simulink model "summerControlledGroup8"  (R2023b)
settings: Solver=VariableStepAuto  StartTime=0.0  StopTime=49860  RelTol=1e-3
undefined symbols (not defined in the file): J, Kd, Ke, Ks, Kt, La, Ra
libraries: slpidlib x2, simulink_extras x1
settings Model: Creator=jmars  LastModifiedBy=jmars
settings DataIOCC: ExternalInput=[dec_time dec_azimuth dec_altitude]  LoadExternalInput=on

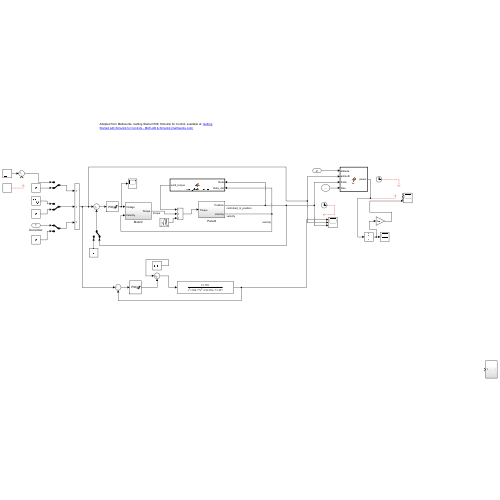
[thumbnail: Simulink's stored preview of the top-level diagram]
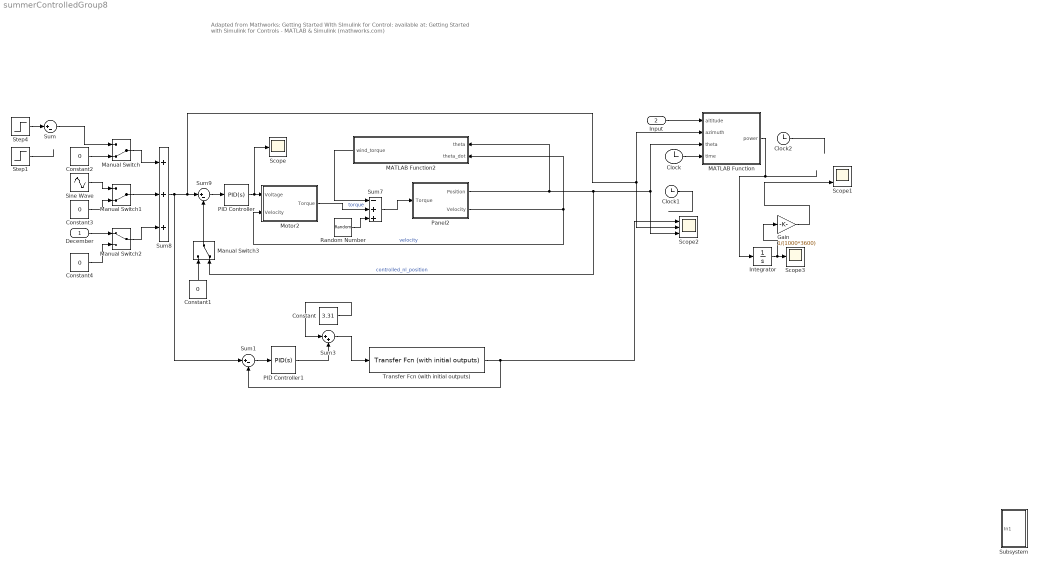
== system summerControlledGroup8 ==
  note: Adapted from Mathworks: Getting Started WIth SImulink for Control: available at: Getting Started with Simulink for Controls - MATLAB & Simulink (mathworks.com)
  December : Inport
  Input : Inport  Port=2
  Clock : Clock
  Clock1 : Clock
  Clock2 : Clock
      settings: Decimation=5
  Constant : Constant  Value=3.31  OutMin=[0]
  Constant{1..4} (4 alike) : Constant  Value=0
  Gain : Gain  Gain=1/(1000*3600)
  Integrator : Integrator
  MATLAB Function : MATLAB Function  TreatAsAtomicUnit=on
  MATLAB Function2 : MATLAB Function  TreatAsAtomicUnit=on
  Manual Switch : ManualSwitch  CurrentSetting=0
  Manual Switch1 : ManualSwitch  CurrentSetting=0
  Manual Switch2 : ManualSwitch
  Manual Switch3 : ManualSwitch  CurrentSetting=0
  Motor2 : Subsystem
  PID Controller : slpidlib/PID Controller  Controller=PID  Form=Parallel  TimeDomain=Continuous-time  UseExternalTs=off  SampleTime=-1  IntegratorMethod=Forward Euler  FilterMethod=Forward Euler  ControllerParametersSource=internal  P=6141/100  I=2.535e4/100  UseKiTs=off  D=4.098e4/100  N=13.7703  UseFilter=on  TunerSelectOption=Transfer Function Based (PID Tuner App)  InitialConditionSource=internal  InitialConditionForIntegrator=0  InitialConditionForFilter=0  DifferentiatorICPrevScaledInput=0  ExternalReset=none  TrackingMode=off  Kt=1  LimitOutput=on  SatLimitsSource=internal  UpperSaturationLimit=27.5  LowerSaturationLimit=-27.5  LinearizeAsGain=on  AntiWindupMode=none  Kb=1  LimitIntegrator=off  UpperIntegratorSaturationLimit=inf  LowerIntegratorSaturationLimit=-inf  POutMin=[]  POutMax=[]  IOutMin=[]  IOutMax=[]  DOutMin=[]  DOutMax=[]  NOutMin=[]  NOutMax=[]  SumOutMin=[]  SumOutMax=[]  SaturationOutMin=[]  SaturationOutMax=[]  PParamMin=[]  PParamMax=[]  IParamMin=[]  IParamMax=[]  DParamMin=[]  DParamMax=[]  NParamMin=[]  NParamMax=[]  KbParamMin=[]  KbParamMax=[]  KtParamMin=[]  KtParamMax=[]  KbOutMin=[]  KbOutMax=[]  KtOutMin=[]  KtOutMax=[]  IntegratorOutMin=[]  IntegratorOutMax=[]  FilterOutMin=[]  FilterOutMax=[]  SumI1OutMin=[]  SumI1OutMax=[]  SumI2OutMin=[]  SumI2OutMax=[]  SumI3OutMin=[]  SumI3OutMax=[]  SumI4OutMin=[]  SumI4OutMax=[]  SumDOutMin=[]  SumDOutMax=[]  DifferentiatorOutMin=[]  DifferentiatorOutMax=[]  FilterDiffOutCoefMin=[]  FilterDiffOutCoefMax=[]  ReciprocalOutMin=[]  ReciprocalOutMax=[]  SumDenOutMin=[]  SumDenOutMax=[]  SumNumOutMin=[]  SumNumOutMax=[]  DivideOutMin=[]  DivideOutMax=[]  UdiffTsProdOutMin=[]  UdiffTsProdOutMax=[]  NTsProdOutMin=[]  NTsProdOutMax=[]  UintegralTsProdOutMin=[]  UintegralTsProdOutMax=[]  UngainTsProdOutMin=[]  UngainTsProdOutMax=[]  ClampingZeroOutDataTypeStr=Inherit: Inherit via back propagation  ClampingZeroOutMin=[]  ClampingZeroOutMax=[]  FilterDenConstantOutDataTypeStr=Inherit: Inherit via back propagation  FilterDenConstantOutMin=[]  FilterDenConstantOutMax=[]  PCopyOutDataTypeStr=Inherit: Inherit via back propagation  PCopyOutMin=[]  PCopyOutMax=[]  NCopyOutDataTypeStr=Inherit: Inherit via back propagation  NCopyOutMin=[]  NCopyOutMax=[]  IntegratorContinuousStateAttributes=''  IntegratorStateMustResolveToSignalObject=off  IntegratorRTWStateStorageClass=Auto  FilterContinuousStateAttributes=''  FilterStateMustResolveToSignalObject=off  FilterRTWStateStorageClass=Auto  ParallelPVariant=InternalParameters  IdealPVariant=Disabled  IVariant=InternalParameters  DVariant=InternalParameters  IntegratorVariant=Continuous  SatVariant=Enabled  AWVariant=Passthrough  PCopyVariant=Disabled  TRVariant=Disabled  FdbkBlocksVariant=Forward  IdealPFdbkVariant=Disabled  SatFdbkVariant=Disabled  DerivativeFilterVariant=ContFilter  NVariant=InternalParameters  NCopyVariant=Disabled  FilterICVariant=InternalICsFilter  IntegratorICVariant=InternalICs  ExternalResetVariant=Disabled  TRSumVariant=Passthrough  SumFdbkVariant=Disabled  SumVariant=Sum_PID  TsampFilterVariant=InternalTs  TsampNgainVariant=Passthrough  TsampIntegralVariant=Disabled_SignalSpec  ExternalSaturationOutDataTypeStr=Inherit: Same as second input
  PID Controller1 : slpidlib/PID Controller  Controller=PID  Form=Parallel  TimeDomain=Continuous-time  UseExternalTs=off  SampleTime=-1  IntegratorMethod=Forward Euler  FilterMethod=Forward Euler  ControllerParametersSource=internal  P=6141/100  I=2.535e4/100  UseKiTs=off  D=4.098e4/100  N=13.7703  UseFilter=on  TunerSelectOption=Transfer Function Based (PID Tuner App)  InitialConditionSource=internal  InitialConditionForIntegrator=0  InitialConditionForFilter=0  DifferentiatorICPrevScaledInput=0  ExternalReset=none  TrackingMode=off  Kt=1  LimitOutput=on  SatLimitsSource=internal  UpperSaturationLimit=27.5  LowerSaturationLimit=-27.5  LinearizeAsGain=on  AntiWindupMode=none  Kb=1  LimitIntegrator=off  UpperIntegratorSaturationLimit=inf  LowerIntegratorSaturationLimit=-inf  POutMin=[]  POutMax=[]  IOutMin=[]  IOutMax=[]  DOutMin=[]  DOutMax=[]  NOutMin=[]  NOutMax=[]  SumOutMin=[]  SumOutMax=[]  SaturationOutMin=[]  SaturationOutMax=[]  PParamMin=[]  PParamMax=[]  IParamMin=[]  IParamMax=[]  DParamMin=[]  DParamMax=[]  NParamMin=[]  NParamMax=[]  KbParamMin=[]  KbParamMax=[]  KtParamMin=[]  KtParamMax=[]  KbOutMin=[]  KbOutMax=[]  KtOutMin=[]  KtOutMax=[]  IntegratorOutMin=[]  IntegratorOutMax=[]  FilterOutMin=[]  FilterOutMax=[]  SumI1OutMin=[]  SumI1OutMax=[]  SumI2OutMin=[]  SumI2OutMax=[]  SumI3OutMin=[]  SumI3OutMax=[]  SumI4OutMin=[]  SumI4OutMax=[]  SumDOutMin=[]  SumDOutMax=[]  DifferentiatorOutMin=[]  DifferentiatorOutMax=[]  FilterDiffOutCoefMin=[]  FilterDiffOutCoefMax=[]  ReciprocalOutMin=[]  ReciprocalOutMax=[]  SumDenOutMin=[]  SumDenOutMax=[]  SumNumOutMin=[]  SumNumOutMax=[]  DivideOutMin=[]  DivideOutMax=[]  UdiffTsProdOutMin=[]  UdiffTsProdOutMax=[]  NTsProdOutMin=[]  NTsProdOutMax=[]  UintegralTsProdOutMin=[]  UintegralTsProdOutMax=[]  UngainTsProdOutMin=[]  UngainTsProdOutMax=[]  ClampingZeroOutDataTypeStr=Inherit: Inherit via back propagation  ClampingZeroOutMin=[]  ClampingZeroOutMax=[]  FilterDenConstantOutDataTypeStr=Inherit: Inherit via back propagation  FilterDenConstantOutMin=[]  FilterDenConstantOutMax=[]  PCopyOutDataTypeStr=Inherit: Inherit via back propagation  PCopyOutMin=[]  PCopyOutMax=[]  NCopyOutDataTypeStr=Inherit: Inherit via back propagation  NCopyOutMin=[]  NCopyOutMax=[]  IntegratorContinuousStateAttributes=''  IntegratorStateMustResolveToSignalObject=off  IntegratorRTWStateStorageClass=Auto  FilterContinuousStateAttributes=''  FilterStateMustResolveToSignalObject=off  FilterRTWStateStorageClass=Auto  ParallelPVariant=InternalParameters  IdealPVariant=Disabled  IVariant=InternalParameters  DVariant=InternalParameters  IntegratorVariant=Continuous  SatVariant=Enabled  AWVariant=Passthrough  PCopyVariant=Disabled  TRVariant=Disabled  FdbkBlocksVariant=Forward  IdealPFdbkVariant=Disabled  SatFdbkVariant=Disabled  DerivativeFilterVariant=ContFilter  NVariant=InternalParameters  NCopyVariant=Disabled  FilterICVariant=InternalICsFilter  IntegratorICVariant=InternalICs  ExternalResetVariant=Disabled  TRSumVariant=Passthrough  SumFdbkVariant=Disabled  SumVariant=Sum_PID  TsampFilterVariant=InternalTs  TsampNgainVariant=Passthrough  TsampIntegralVariant=Disabled_SignalSpec  ExternalSaturationOutDataTypeStr=Inherit: Same as second input
  Panel2 : Subsystem
  Random Number : RandomNumber  Variance=0.01  SampleTime=10
  Scope : Scope
  Scope1 : Scope  NumInputPorts=3
  Scope2 : Scope  NumInputPorts=3
  Scope3 : Scope
  Sine Wave : Sin  Bias=1.1019  SampleTime=0
  Step1 : Step  Time=20  After=8.8981  SampleTime=0
  Step4 : Step  Time=10  Before=1.1019  After=10  SampleTime=0
  Subsystem : Subsystem
  Sum : Sum  Inputs=|+-
  Sum1 : Sum  Inputs=|+-
  Sum3 : Sum  Inputs=|++
  Sum7 : Sum  Inputs=-++
  Sum8 : Sum  Inputs=+++
  Sum9 : Sum  Inputs=|+-
  Transfer Fcn (with initial outputs) : simulink_extras/Additional Linear/Transfer Fcn (with initial outputs)  N=[23.7894]  D="[1  306.7708 182.0498 71.4275]"  Y0=1.1019  U0=3.31
  wires:
  Sine Wave/1 -> Manual Switch1/1
  Manual Switch2/1 -> Sum8/3
  Manual Switch1/1 -> Sum8/2
  Constant4/1 -> Manual Switch2/2
  Panel2/1(Position) -> Manual Switch3/2, Scope2/3, MATLAB Function/3(theta), MATLAB Function2/1(theta)  "controlled_nl_position"
  Sum7/1 -> Panel2/1(Torque)
  Sum8/1 -> Sum1/1, Scope2/2, MATLAB Function/2(azimuth), Sum9/1
  December/1 -> Manual Switch2/1
  Constant2/1 -> Manual Switch/2
  Sum9/1 -> PID Controller/1
  Manual Switch/1 -> Sum8/1
  Motor2/1(Torque) -> Sum7/2  "torque"
  Constant3/1 -> Manual Switch1/2
  MATLAB Function2/1(wind_torque) -> Sum7/1
  Panel2/2(Velocity) -> Motor2/2(Velocity), MATLAB Function2/2(theta_dot)  "velocity"
  Step4/1 -> Sum/1
  Sum/1 -> Manual Switch/1
  Step1/1 -> ?
  Manual Switch3/1 -> Sum9/2
  Constant1/1 -> Manual Switch3/1
  Sum1/1 -> PID Controller1/1
  Transfer Fcn (with initial outputs)/1 -> Scope2/1, Sum1/2
  PID Controller/1 -> Scope/1, Motor2/1(Voltage)
  Random Number/1 -> Sum7/3
  Input/1 -> MATLAB Function/1(altitude)
  Clock/1 -> MATLAB Function/4(time)
  MATLAB Function/1(power) -> Integrator/1
  Integrator/1 -> Gain/1, Scope3/1
  PID Controller1/1 -> Sum3/2
  Constant/1 -> Sum3/1
  Sum3/1 -> Transfer Fcn (with initial outputs)/1
  Clock1/1 -> ?
  Gain/1 -> Scope1/3
  Clock2/1 -> ?

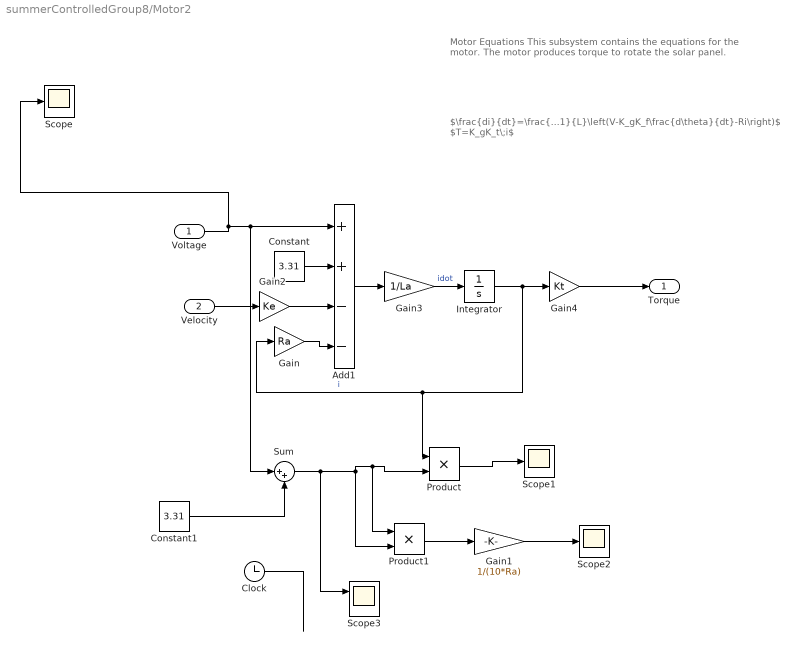
== system summerControlledGroup8/Motor2 ==
  note: $\frac{di}{dt}=\frac{1}{L}\left(V-K_gK_f\frac{d\theta}{dt}-Ri\right)$
      | $T=K_gK_t\;i$
  note: Motor Equations
      |
      | This subsystem contains the equations for the motor. The motor produces torque to rotate the solar panel.
  Voltage : Inport
  Velocity : Inport  Port=2
  Add1 : Sum  Inputs=++--
  Clock : Clock
      settings: Decimation=5
  Constant : Constant  Value=3.31  OutMin=[0]
  Constant1 : Constant  Value=3.31  OutMin=[0]
  Gain : Gain  Gain=Ra
  Gain1 : Gain  Gain=1/(10*Ra)
  Gain2 : Gain  Gain=Ke
  Gain3 : Gain  Gain=1/La
  Gain4 : Gain  Gain=Kt
  Integrator : Integrator  InitialCondition=3.5
  Product : Product
  Product1 : Product
  Scope : Scope
  Scope1 : Scope
  Scope2 : Scope
  Scope3 : Scope  NumInputPorts=2
  Sum : Sum  Inputs=|++
  Torque : Outport
  wires:
  Voltage/1 -> Scope/1, Sum/1, Add1/1
  Gain2/1 -> Add1/3
  Gain3/1 -> Integrator/1  "idot"
  Gain/1 -> Add1/4
  Integrator/1 -> Product/1, Gain/1, Gain4/1  "i"
  Add1/1 -> Gain3/1
  Velocity/1 -> Gain2/1
  Gain4/1 -> Torque/1
  Constant/1 -> Add1/2
  Product/1 -> Scope1/1
  Sum/1 -> Scope3/1, Product1/1, Product/2, Product1/2
  Constant1/1 -> Sum/2
  Product1/1 -> Gain1/1
  Gain1/1 -> Scope2/1
  Clock/1 -> ?

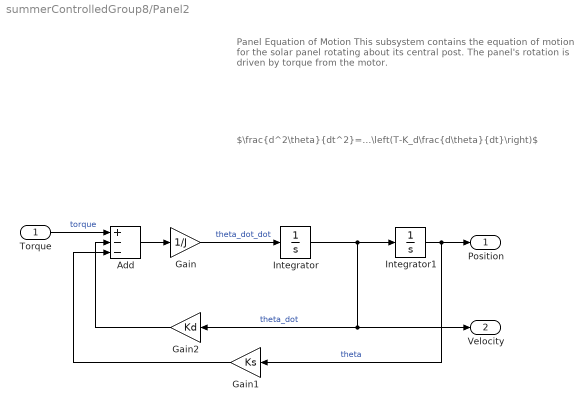
== system summerControlledGroup8/Panel2 ==
  note: $\frac{d^2\theta}{dt^2}=\frac{1}{J}\left(T-K_d\frac{d\theta}{dt}\right)$
  note: Panel Equation of Motion
      |
      | This subsystem contains the equation of motion for the solar panel rotating about its central post. The panel's rotation is driven by torque from the motor.
  Torque : Inport
  Add : Sum  Inputs=+--
  Gain : Gain  Gain=1/J
  Gain1 : Gain  Gain=Ks
  Gain2 : Gain  Gain=Kd
  Integrator : Integrator
  Integrator1 : Integrator  InitialCondition=1.1019
  Position : Outport
  Velocity : Outport  Port=2
  wires:
  Torque/1 -> Add/1  "torque"
  Add/1 -> Gain/1
  Integrator/1 -> Velocity/1, Gain2/1, Integrator1/1  "theta_dot"
  Gain2/1 -> Add/2
  Gain/1 -> Integrator/1  "theta_dot_dot"
  Integrator1/1 -> Gain1/1, Position/1  "theta"
  Gain1/1 -> Add/3

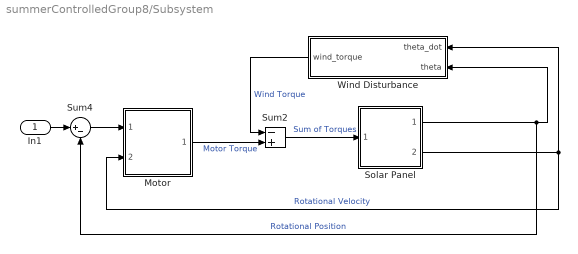
== system summerControlledGroup8/Subsystem ==
  In1 : Inport
  Motor : Subsystem
      mask Display: image('motor.png');
  Solar Panel : Subsystem
      mask Display: image('panel.png');
  Sum2 : Sum  Inputs=-+
  Sum4 : Sum  Inputs=|+-
  Wind Disturbance : MATLAB Function  TreatAsAtomicUnit=on
  wires:
  Solar Panel/1(Rotational Position) -> Wind Disturbance/2(theta), Sum4/2  "Rotational Position"
  Sum2/1 -> Solar Panel/1(External Torques)  "Sum of Torques"
  Solar Panel/2(Rotational Velocity) -> Motor/2(Rotational Velocity), Wind Disturbance/1(theta_dot)  "Rotational Velocity"
  In1/1 -> Sum4/1
  Wind Disturbance/1(wind_torque) -> Sum2/1  "Wind Torque"
  Motor/1(Motor Torque) -> Sum2/2  "Motor Torque"
  Sum4/1 -> Motor/1(Voltage)

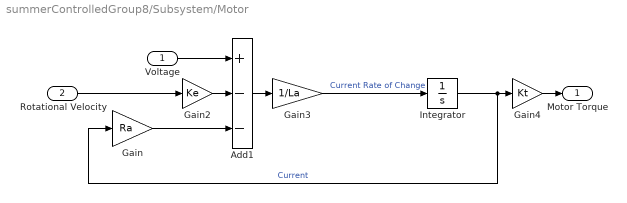
== system summerControlledGroup8/Subsystem/Motor ==
  Voltage : Inport
  Rotational Velocity : Inport  Port=2
  Add1 : Sum  Inputs=+--
  Gain : Gain  Gain=Ra
  Gain2 : Gain  Gain=Ke
  Gain3 : Gain  Gain=1/La
  Gain4 : Gain  Gain=Kt
  Integrator : Integrator
  Motor Torque : Outport
  wires:
  Voltage/1 -> Add1/1
  Gain2/1 -> Add1/2
  Gain3/1 -> Integrator/1  "Current Rate of Change"
  Gain/1 -> Add1/3
  Integrator/1 -> Gain4/1, Gain/1  "Current"
  Add1/1 -> Gain3/1
  Rotational Velocity/1 -> Gain2/1
  Gain4/1 -> Motor Torque/1

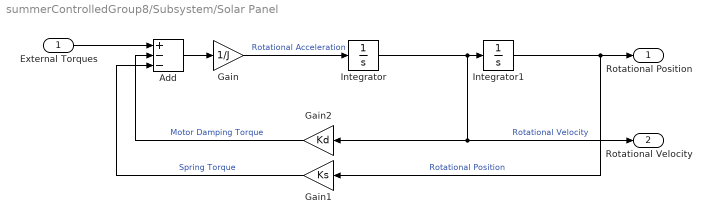
== system summerControlledGroup8/Subsystem/Solar Panel ==
  External Torques : Inport
  Add : Sum  Inputs=+--
  Gain : Gain  Gain=1/J
  Gain1 : Gain  Gain=Ks
  Gain2 : Gain  Gain=Kd
  Integrator : Integrator
  Integrator1 : Integrator
  Rotational Position : Outport
  Rotational Velocity : Outport  Port=2
  wires:
  External Torques/1 -> Add/1
  Add/1 -> Gain/1
  Integrator/1 -> Integrator1/1, Rotational Velocity/1, Gain2/1  "Rotational Velocity"
  Gain2/1 -> Add/2  "Motor Damping Torque"
  Gain/1 -> Integrator/1  "Rotational Acceleration"
  Integrator1/1 -> Gain1/1, Rotational Position/1  "Rotational Position"
  Gain1/1 -> Add/3  "Spring Torque"

== matlab function summerControlledGroup8/Subsystem/Wind Disturbance ==
  data: theta_dot input; theta input; wind_torque output
function wind_torque = wind_disturbance(theta_dot, theta)
%Wind
w = 1.134; % Width, [m]
l = 2.279; % Length, [m]
U = 3.6; %Wind Speed
rho = 1.09; %Density 
Cd = 1.17; % Drag Coefficient
r = 0.5*w; 

wind_torque = abs(2/3*rho*Cd*l*U*sind(30)*sin(theta)*theta_dot*r^3);

== matlab function summerControlledGroup8/MATLAB Function ==
  data: altitude input; power output; azimuth input; theta input; time input
function power = fcn(altitude, azimuth, theta, time)
eff = 0.228;
%irr = -4e-24*time^6 + 7e-19*time^5 -4e-14*time^4 +9e-10*time^3 -6e-06*time^2 +0.0125*time +20.724;
%irr=time^2 + 1
%t=;

x = [0 3600 7200 10800 14400 18000 21600 25200 28800 32400 36000 39600 43200 46800 50400];
y = [10 40.0195122 71.46341463 110.0536585 383.0439024 624.5902439 800.3902439 893.2926829 894.7219512 806.1073171 634.595122 394.4780488 121.4878049 65 0];
%xx = 0:3600:50400;
irr = spline(x,y,time);
power = irr * eff *  sin((pi/6)+altitude)*(1-abs((theta-azimuth)/azimuth));

== matlab function summerControlledGroup8/MATLAB Function2 ==
  data: theta input; wind_torque output; theta_dot input
function wind_torque = wind_disturbance(theta, theta_dot)
%Wind
w = 1.134; % Width, [m]
l = 2.279; % Length, [m]
U = 3.6; %Wind Speed
rho = 1.09; %Density 
Cd = 1.17; % Drag Coefficient
r = 0.5*w; 

wind_torque = abs(2/3*rho*Cd*l*U*sind(30)*sin(theta)*theta_dot*r^3);
